simulink model "gm_pmsm_fpga_slrt"  (R2020b)
settings: Solver=FixedStepDiscrete  StartTime=0.0  StopTime=5  FixedStep=1e-5  RelTol=1e-3
PostLoadFcn:
  | try
  | cell = struct2cell(dir(fullfile(speedgoatroot_hdlb, 'hdlsrc', 'pwm', '*.vhd')));
  | addSourceFiles = strjoin(fullfile(cell(2,:),cell(1,:)), ';');
  | hdlset_param('pwm_example_hdlc/DUT PWM and CAP', 'IPCoreAdditionalFiles', addSourceFiles);
  | end
InitFcn:
  | Ts=50e-6;     %simulation time step
  | kp = 1e-4;   %proportional gain
  | ki =0.01e-1;     %integral gain
  | fsw = 1e3;     %switching frequency
undefined symbols (not defined in the file): DiscIntNeverNeededParam, FPGA, IO334, pmsm_fpga
libraries: speedgoatlib_hdlCoder_IO3xx x11, powerlib x9, powerlib_meascontrol x6, quadrature_cpulib x1, slrealtimeutilitieslib x1, pwm_cpulib x1, eeQuadratureDecoder x1, simulink x1, mcbplantlib x1
settings Model: ModifiedByFormat=Speedgoat GmbH  SimulationMode=external  Creator=Speedgoat GmbH  LastModifiedBy=Speedgoat GmbH
settings SolverCC: ConcurrentTasks=on  PositivePriorityOrder=on
settings DataIOCC: LimitDataPoints=on  SaveFormat=Array  ReturnWorkspaceOutputs=off
settings OptimizationCC: BlockReduction=off  ConditionallyExecuteInputs=off  DefaultParameterBehavior=Inlined  OptimizeBlockIOStorage=off
settings DebuggingCC: AlgebraicLoopMsg=error  UnderspecifiedInitializationDetection=Classic  MergeDetectMultiDrivingBlocksExec=none  SolverPrmCheckMsg=warning  InheritedTsInSrcMsg=none  SingleTaskRateTransMsg=error  TasksWithSamePriorityMsg=none  ParameterPrecisionLossMsg=none  PregeneratedLibrarySubsystemCodeDiagnostic=none  SFUnexpectedBacktrackingDiag=warning  SFNoUnconditionalDefaultTransitionDiag=warning  SFExecutionAtInitializationDiag=none  ArithmeticOperatorsInVariantConditions=warning
settings HardwareCC: ProdBitPerLong=64  ProdLongLongMode=on  ProdHWDeviceType=Intel->x86-64 (Linux 64)
settings ModelReferenceCC: PropagateSignalLabelsOutOfModel=off
settings SFSimCC: SimUseLocalCustomCode=off  CustomCodeUndefinedFunction=UseInterfaceOnly
settings RTWCC: Description=Simulink Real-Time  SystemTargetFile=slrealtime.tlc  TemplateMakefile=slrealtime_default_tmf  RTWUseLocalCustomCode=off  Toolchain=Simulink Real-Time Toolchain  BuildConfiguration=Faster Runs  CodeExecutionProfiling=on  TargetLang=C++
settings CodeAppCC: StateflowObjectComments=on
settings ConfigComp: CovMetricSettings=dw  CovSaveCumulativeToWorkspaceVar=on  CovSaveSingleToWorkspaceVar=on  CovExternalEMLEnable=off

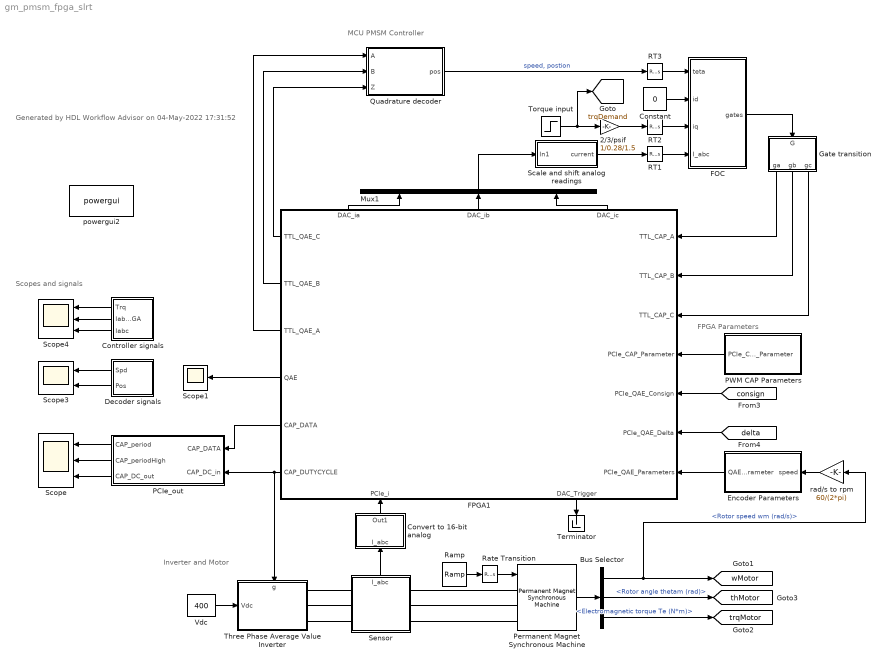
== system gm_pmsm_fpga_slrt ==
  note: Generated by HDL Workflow Advisor on 04-May-2022 17:31:52
  note: FPGA Parameters
  note: Inverter and Motor
  note: MCU PMSM Controller
  note: Scopes and signals
  2/3/psif : Gain  Gain=1/0.28/1.5  SaturateOnIntegerOverflow=on  OutDataTypeStr=Inherit: Same as input  ParamDataTypeStr=Inherit: Same as input
  Bus Selector : BusSelector  OutputSignals=Rotor speed wm (rad/s),Rotor angle thetam (rad),Electromagnetic torque Te (N*m)
  Constant : Constant  Value=0  SampleTime=-1
  Controller signals : Subsystem
  Convert to 16-bit analog : Subsystem
  Decoder signals : Subsystem
  Encoder Parameters : Subsystem
  FOC : Subsystem
  FPGA1 : Subsystem  mask(Speedgoat IO334-325k Interface Block){module_id=1, slot=-1, ts=-1, OutputRange=Auto (same as ADC), PullRPort0=pull-up 3.3V, VioPort0=3.3V, PullRPort1=pull-up 3.3V, VioPort1=3.3V, PullRPort2=pull-up 3.3V, VioPort2=3.3V, PullRPort3=pull-up 3.3V, VioPort3=3.3V, PullRPort4=pull-up 3.3V, VioPort4=3.3V, PullRPort5=pull-up 3.3V, VioPort5=3.3V, PullRPort6=pull-up 3.3V, VioPort6=3.3V, FpgaFreq=100}
      mask prompts: module_id "FPGA Module Identifier:"; slot "PCI slot (-1: autosearch):"; ts "Sample time:"; OutputRange "DAC Voltage Range:"; PullRPort0 "pull resistor"; VioPort0 "I/O voltage"; PullRPort1 "pull resistor"; VioPort1 "I/O voltage"; PullRPort2 "pull resistor"; VioPort2 "I/O voltage"; PullRPort3 "pull resistor"; VioPort3 "I/O voltage"; PullRPort4 "pull resistor"; VioPort4 "I/O voltage"; PullRPort5 "pull resistor"; VioPort5 "I/O voltage"; PullRPort6 "pull resistor"; VioPort6 "I/O voltage"; FpgaFreq "FPGA Frequency [MHz]"
      mask help: Simulink Real-Time Interface Block for Speedgoat IO334-325k.
      mask init:
      | hdlslrt.backend.mfpgaparameters;
      settings: PortSchema="{\"entries\":[{\"content\":{\"sides\":[{\"content\":{\"connectorIds\":[\"Out5\",\"Out6\",\"Out7\",\"Out8\",\"Out9\",\"Out10\"]},\"type\":\"ConnectorPlacement.EquallySpacedRectSide\",\"uuid\":\"34ddc533-e92e-4f84-ab54-56ee31c34ed5\"},{\"content\":{\"connectorIds\":[\"In2\",\"In3\",\"In4\",\"In5\",\"In6\",\"In7\",\"In8\"],\"side\":\"RIGHT\"},\"type\":\"ConnectorPlacement.EquallySpacedRectSide\",\"uuid\":\"fc43732f-8b85-47c9-af73-b87840a05fb5\"},{\"content\":{\"connectorIds\":[\"Out2\",\"Out3\",\"Out4\"],\"side\":\"TOP\"},\"type\":\"ConnectorPlacement.EquallySpacedRectSide\",\"uuid\":\"bf663b9c-33b6-4726-afdb-56df835214b8\"},{\"content\":{\"connectorIds\":[\"In1\",\"Out1\"],\"side\":\"BOTTOM\"},\"type\":\"ConnectorPlacement.EquallySpacedRectSide\",\"uuid\":\"04fbffa8-14ef-4425-a219-a420a37a7cbf\"},{\"content\":{\"connectorIds\":[],\"side\":\"HIDDEN\"},\"type\":\"ConnectorPlacement.EquallySpacedRectSide\",\"uuid\":\"ed9b2637-afe7-435a-b994-99eac90c9c32\"}]},\"type\":\"ConnectorPlacement.EquallySpacedConnector\",\"uuid\":\"b4b9272a-3f4d-4e79-a573-4a3ad4933ba9\"}],\"packageUris\":[\"http://schema.mathworks.com/mf0/Connector/R2020b\"],\"version\":\"1.0\"}"
      mask Help: eval('speedgoatdoc_hdlc')
      mask TypeOptions OutputRange: IO334 DAC Setup/OutputRange
      mask TypeOptions PullRPort0: Port Settings -2x/PullRPort0
      mask Callback PullRPort0: sg_fpga_HDLCoder_io3xx_2x_m(2)
      mask TypeOptions VioPort0: Port Settings -2x/VioPort0
      mask Callback VioPort0: sg_fpga_HDLCoder_io3xx_2x_m(2)
      mask TypeOptions PullRPort1: Port Settings -2x/PullRPort1
      mask Callback PullRPort1: sg_fpga_HDLCoder_io3xx_2x_m(2)
      mask TypeOptions VioPort1: Port Settings -2x/VioPort1
      mask Callback VioPort1: sg_fpga_HDLCoder_io3xx_2x_m(2)
      mask TypeOptions PullRPort2: Port Settings -2x/PullRPort2
      mask Callback PullRPort2: sg_fpga_HDLCoder_io3xx_2x_m(2)
      mask TypeOptions VioPort2: Port Settings -2x/VioPort2
      mask Callback VioPort2: sg_fpga_HDLCoder_io3xx_2x_m(2)
      mask TypeOptions PullRPort3: Port Settings -2x/PullRPort3
      mask Callback PullRPort3: sg_fpga_HDLCoder_io3xx_2x_m(2)
      mask TypeOptions VioPort3: Port Settings -2x/VioPort3
      mask Callback VioPort3: sg_fpga_HDLCoder_io3xx_2x_m(2)
      mask TypeOptions PullRPort4: Port Settings -2x/PullRPort4
      mask Callback PullRPort4: sg_fpga_HDLCoder_io3xx_2x_m(2)
      mask TypeOptions VioPort4: Port Settings -2x/VioPort4
      mask Callback VioPort4: sg_fpga_HDLCoder_io3xx_2x_m(2)
      mask TypeOptions PullRPort5: Port Settings -2x/PullRPort5
      mask Callback PullRPort5: sg_fpga_HDLCoder_io3xx_2x_m(2)
      mask TypeOptions VioPort5: Port Settings -2x/VioPort5
      mask Callback VioPort5: sg_fpga_HDLCoder_io3xx_2x_m(2)
      mask TypeOptions PullRPort6: Port Settings -2x/PullRPort6
      mask Callback PullRPort6: sg_fpga_HDLCoder_io3xx_2x_m(2)
      mask TypeOptions VioPort6: Port Settings -2x/VioPort6
      mask Callback VioPort6: sg_fpga_HDLCoder_io3xx_2x_m(2)
      mask DialogControl AnalogOutput Prompt: Analog Output
      mask DialogControl IO33421 Prompt: IO334-21
      mask DialogControl port1 Prompt: Port 1
      mask DialogControl port2 Prompt: Port 2
      mask DialogControl port3 Prompt: Port 3
      mask DialogControl port4 Prompt: Port 4
      mask DialogControl port5 Prompt: Port 5
      mask DialogControl port6 Prompt: Port 6
      mask DialogControl port7 Prompt: Port 7
      mask Display:
      | SetupBlkPath = find_system(gcb, 'LookUnderMasks', 'all', 'FollowLinks', 'on', 'regexp', 'on', 'Name', 'IO3(\d|x){2}\s+Setup' );
      | SetupBlkPath = SetupBlkPath{1};
      | TS = get_param(SetupBlkPath,'timestamp_mcs');
      | disp(sprintf('Speedgoat IO334-325k\nFPGA I/O Module\n\nTimestamp\n%s\n\nReference Design\nVersion 2.1\n\nMatlab R2020b\n\nPCIe Link Width: X4\nRear Plugin: -21\nAurora Mode: None\nAurora Byteswap: true\n', TS))
  Gate transition : Subsystem
  Mux1 : Mux  Inputs=3
  PCIe_out : Subsystem
  PWM CAP Parameters : Subsystem
  Permanent Magnet Synchronous Machine : powerlib/Machines/Permanent Magnet Synchronous Machine  NbPhases=3  FluxDistribution=Sinusoidal  RotorType=Salient-pole  MechanicalLoad=Speed w  PresetModel=No  ShowDetailedParameters=on  MeasurementBus=off  Resistance=0.1  Inductance=8.5e-3  dqInductances="[0.00006  0.00008]*10"  La=0.000395  MachineConstant=Flux linkage established by magnets (V.s)  Flux=0.28  VoltageCst=50.7864  TorqueCst=0.42  Flat=120  Mechanical=[0.0027 0.0004924 1 0]  PolePairs=1  InitialConditions=[0,0, 0,0]  InitialConditions5ph=[0 0 0 0 0 0]  RefAngle=90 degrees behind phase A axis (modified Park)  IterativeDiscreteModel=Trapezoidal non iterative  TsBlock=-1  TsPowergui=0
  Quadrature decoder : Subsystem
  RT1 : RateTransition  OutPortSampleTimeOpt=Inherit  OutPortSampleTime=Ts
  RT2 : RateTransition  OutPortSampleTimeOpt=Inherit  OutPortSampleTime=Ts
  RT3 : RateTransition  OutPortSampleTimeOpt=Inherit  OutPortSampleTime=Ts
  Ramp : simulink/Sources/Ramp  slope=100/2/60*2*pi  start=0  InitialOutput=0
  Rate Transition : RateTransition  OutPortSampleTime=Ts
  Scale and shift analog readings : Subsystem
  Scope : Scope  NumInputPorts=3
  Scope1 : Scope
  Scope3 : Scope  NumInputPorts=2
  Scope4 : Scope  NumInputPorts=3
  Sensor : Subsystem
      settings: PortSchema="{\"entries\":[{\"content\":{\"sides\":[{\"content\":{\"connectorIds\":[\"LConn1\",\"LConn2\",\"LConn3\"]},\"type\":\"ConnectorPlacement.EquallySpacedRectSide\",\"uuid\":\"d3673cf9-f798-4f95-832a-0ee38b3b4235\"},{\"content\":{\"connectorIds\":[\"RConn1\",\"RConn2\",\"RConn3\"],\"side\":\"RIGHT\"},\"type\":\"ConnectorPlacement.EquallySpacedRectSide\",\"uuid\":\"f1c3e6c7-7356-4e8b-bcca-414f2c82a0be\"},{\"content\":{\"connectorIds\":[\"Out1\"],\"side\":\"TOP\"},\"type\":\"ConnectorPlacement.EquallySpacedRectSide\",\"uuid\":\"10e31bf8-a182-46d8-beca-1ec9bb9081e0\"},{\"content\":{\"connectorIds\":[],\"side\":\"HIDDEN\"},\"type\":\"ConnectorPlacement.EquallySpacedRectSide\",\"uuid\":\"21150a95-24d3-4ba1-92b8-5619804d049c\"}]},\"type\":\"ConnectorPlacement.EquallySpacedConnector\",\"uuid\":\"db0d9e3c-2d98-4024-a8e1-7fc9e86b9a02\"}],\"packageUris\":[\"http://schema.mathworks.com/mf0/Connector/R2020b\"],\"version\":\"1.0\"}"
  Terminator : Terminator
  Three Phase Average Value Inverter : Subsystem
      settings: PortSchema="{\"entries\":[{\"content\":{\"sides\":[{\"content\":{\"connectorIds\":[\"In1\"]},\"type\":\"ConnectorPlacement.EquallySpacedRectSide\",\"uuid\":\"bfacb710-2d3a-4e7b-9063-25c8b87226b9\"},{\"content\":{\"connectorIds\":[\"RConn1\",\"RConn2\",\"RConn3\"],\"side\":\"RIGHT\"},\"type\":\"ConnectorPlacement.EquallySpacedRectSide\",\"uuid\":\"a8d38f79-eb95-4afe-ba2f-2842c1cba801\"},{\"content\":{\"connectorIds\":[\"In2\"],\"side\":\"TOP\"},\"type\":\"ConnectorPlacement.EquallySpacedRectSide\",\"uuid\":\"291d9d52-08e6-4456-8afe-095013b7df64\"},{\"content\":{\"connectorIds\":[],\"side\":\"HIDDEN\"},\"type\":\"ConnectorPlacement.EquallySpacedRectSide\",\"uuid\":\"61aa80b0-9b99-474b-ab67-e014373e5595\"}]},\"type\":\"ConnectorPlacement.EquallySpacedConnector\",\"uuid\":\"1232c420-125a-43af-99e1-be04cd6c95a4\"}],\"packageUris\":[\"http://schema.mathworks.com/mf0/Connector/R2020b\"],\"version\":\"1.0\"}"
  Torque input : Step  Time=0.3  After=300  SampleTime=Ts
  Vdc : Constant  Value=400  SampleTime=Ts
  powergui2 : powerlib/powergui  Priority=1  SimulationMode=Discrete  SampleTime=Ts  frequency=60  Iterations=50  frequencyindice=0  Pbase=100e6  ErrMax=1e-4  UnitsV=kV  UnitsW=MW  buscounter=0  FunctionMessages=off  echomessages=off  EnableUseOfTLC=off  CurrentSourceSwitches=off  DisableSnubberDevices=off  DisableRonSwitches=off  DisableVfSwitches=off  DisplayEquations=off  AutomaticDiscreteSolvers=off  SolverType=Tustin/Backward Euler (TBE)  Interpol=off  ExternalGateDelay=off  methode=off  Ts=100  x0status=blocks  SPID=on  SwTol=0  HookPort=off  NonlinearTolerance=1e-4  nMaxIteration=100  ContinueOnMaxIteration=off  RestoreLinks=warning  ResistiveCurrentMeasurement=off  Frange=[0:2:500]  Ylog=off  Xlog=on  ShowGrid=off  save=off  variable=ZData  structure=0  ZoomFFT=off  StartTime=0.0  cycles=1  DisplayStyle=1  fundamental=60  FreqAxis=off  MaxFrequency=1000  frequencyindicesteady=1  RmsSteady=1  display=off
  rad/s to rpm : Gain  Gain=60/(2*pi)
  tag scope: thMotor=global, trqDemand=global, trqMotor=global, wMotor=global
  wires:
  RT3/1 -> FOC/1(teta)
  Bus Selector/3 -> [trqMotor]  "<Electromagnetic torque Te (N*m)>"
  FPGA1/10(CAP_DUTYCYCLE) -> PCIe_out/2(CAP_DC_in), Three Phase Average Value Inverter/2(g)
  FPGA1/7(TTL_QAE_A) -> Quadrature decoder/1(A)
  Ramp/1 -> Rate Transition/1
  PCIe_out/1(CAP_period) -> Scope/1
  Bus Selector/2 -> [thMotor]  "<Rotor angle thetam (rad)>"
  RT1/1 -> FOC/4(I_abc)
  Bus Selector/1 -> rad/s to rpm/1, [wMotor]  "<Rotor speed wm (rad/s)>"
  FPGA1/8(QAE) -> Scope1/1
  Controller signals/2(Iabc_FPGA) -> Scope4/2
  Scale and shift analog readings/1(current) -> RT1/1
  Controller signals/1(Trq) -> Scope4/1
  Decoder signals/1(Spd) -> Scope3/1
  Sensor/1(I_abc) -> Convert to 16-bit analog/1(I_abc)
  RT2/1 -> FOC/3(iq)
  PCIe_out/3(CAP_DC_out) -> Scope/3
  Permanent Magnet Synchronous Machine/1 -> Bus Selector/1
  Torque input/1 -> [trqDemand], 2/3/psif/1
  Convert to 16-bit analog/1(Out1) -> FPGA1/1(PCIe_i)
  FPGA1/3(DAC_ib) -> Mux1/2
  [consign] -> FPGA1/6(PCIe_QAE_Consign)
  FOC/1(gates) -> Gate transition/1(G)
  FPGA1/1(DAC_Trigger) -> Terminator/1
  Mux1/1 -> Scale and shift analog readings/1(In1)
  FPGA1/2(DAC_ia) -> Mux1/1
  [delta] -> FPGA1/7(PCIe_QAE_Delta)
  Constant/1 -> FOC/2(id)
  Gate transition/1(ga) -> FPGA1/2(TTL_CAP_A)
  Vdc/1 -> Three Phase Average Value Inverter/1(Vdc)
  FPGA1/4(DAC_ic) -> Mux1/3
  Controller signals/3(Iabc) -> Scope4/3
  Decoder signals/2(Pos) -> Scope3/2
  Gate transition/2(gb) -> FPGA1/3(TTL_CAP_B)
  FPGA1/6(TTL_QAE_B) -> Quadrature decoder/2(B)
  2/3/psif/1 -> RT2/1
  Quadrature decoder/1(pos) -> RT3/1  "speed, postion"
  Encoder Parameters/1(QAE_parameter) -> FPGA1/8(PCIe_QAE_Parameters)
  FPGA1/5(TTL_QAE_C) -> Quadrature decoder/3(Z)
  PCIe_out/2(CAP_periodHigh) -> Scope/2
  PWM CAP Parameters/1(PCIe_CAP_Parameter) -> FPGA1/5(PCIe_CAP_Parameter)
  rad/s to rpm/1 -> Encoder Parameters/1(speed)
  FPGA1/9(CAP_DATA) -> PCIe_out/1(CAP_DATA)
  Gate transition/3(gc) -> FPGA1/4(TTL_CAP_C)
  Rate Transition/1 -> Permanent Magnet Synchronous Machine/1
  connections:
  Sensor/LConn3 -- Three Phase Average Value Inverter/RConn3
  Permanent Magnet Synchronous Machine/LConn1 -- Sensor/RConn1
  Sensor/LConn2 -- Three Phase Average Value Inverter/RConn2
  Sensor/LConn1 -- Three Phase Average Value Inverter/RConn1
  Permanent Magnet Synchronous Machine/LConn2 -- Sensor/RConn2
  Permanent Magnet Synchronous Machine/LConn3 -- Sensor/RConn3

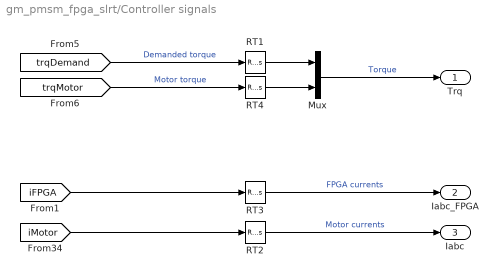
== system gm_pmsm_fpga_slrt/Controller signals ==
  Mux : Mux  Inputs=2
  RT{1..4} (4 alike) : RateTransition  OutPortSampleTime=Ts
  Trq : Outport  VectorParamsAs1DForOutWhenUnconnected=off
  Iabc_FPGA : Outport  Port=2  VectorParamsAs1DForOutWhenUnconnected=off
  Iabc : Outport  Port=3  VectorParamsAs1DForOutWhenUnconnected=off
  wires:
  RT4/1 -> Mux/2
  [trqMotor] -> RT4/1  "Motor torque"
  Mux/1 -> Trq/1  "Torque"
  [iFPGA] -> RT3/1
  RT2/1 -> Iabc/1  "Motor currents"
  [iMotor] -> RT2/1
  RT3/1 -> Iabc_FPGA/1  "FPGA currents"
  RT1/1 -> Mux/1
  [trqDemand] -> RT1/1  "Demanded torque"

== system gm_pmsm_fpga_slrt/Convert to 16-bit analog ==
  I_abc : Inport
  1-D Lookup Table : Lookup_n-D  NumberOfTableDimensions=1  BreakpointsForDimension1=[-2^15, 2^15]  Table=[0, 3.3/10*(2^15-1)]  InternalRulePriority=Speed  RndMeth=Simplest  InputSameDT=on
  Data Type Conversion : DataTypeConversion  OutDataTypeStr=int16
  Gain : Gain  Gain=2^3
  Out1 : Outport
  wires:
  Gain/1 -> 1-D Lookup Table/1
  I_abc/1 -> Gain/1
  1-D Lookup Table/1 -> Data Type Conversion/1
  Data Type Conversion/1 -> Out1/1

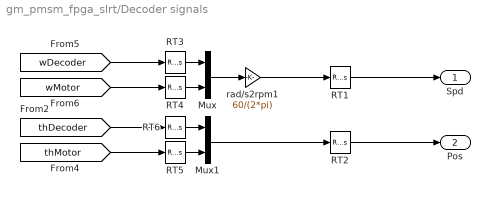
== system gm_pmsm_fpga_slrt/Decoder signals ==
  Mux : Mux  Inputs=2
  Mux1 : Mux  Inputs=2
  RT{1..6} (6 alike) : RateTransition  OutPortSampleTime=Ts
  rad/s2rpm1 : Gain  Gain=60/(2*pi)
  Spd : Outport  VectorParamsAs1DForOutWhenUnconnected=off
  Pos : Outport  Port=2  VectorParamsAs1DForOutWhenUnconnected=off
  wires:
  RT6/1 -> Mux1/1
  RT3/1 -> Mux/1
  rad/s2rpm1/1 -> RT1/1
  RT5/1 -> Mux1/2
  RT4/1 -> Mux/2
  RT2/1 -> Pos/1
  RT1/1 -> Spd/1
  [thMotor] -> RT5/1
  [wMotor] -> RT4/1
  Mux1/1 -> RT2/1
  [thDecoder] -> RT6/1
  Mux/1 -> rad/s2rpm1/1
  [wDecoder] -> RT3/1

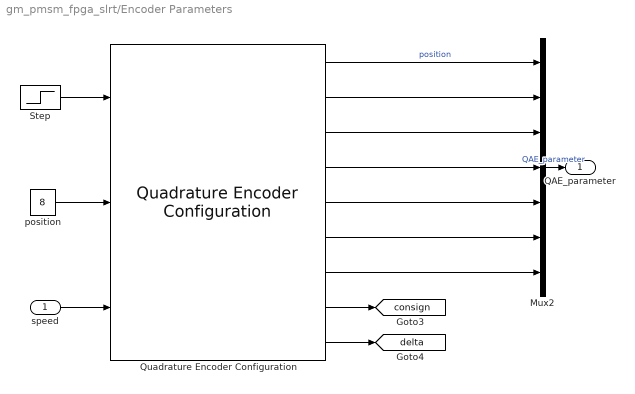
== system gm_pmsm_fpga_slrt/Encoder Parameters ==
  speed : Inport
  Mux2 : Mux  Inputs=7
  Quadrature Encoder Configuration : quadrature_cpulib/Quadrature Encoder Configuration  fpgaFreq=100e6  n_channels=1  numSeg=[512]  phaseAngle=90  initPos=[0]  freeWheel=on
      settings: SourceProductName=Simulink Real-Time: Speedgoat HDL Blockset
  Step : Step  Time=0.002
  position : Constant  Value=8  SampleTime=-1
  QAE_parameter : Outport
  tag scope: consign=global, delta=global
  wires:
  Quadrature Encoder Configuration/3 -> Mux2/3
  Quadrature Encoder Configuration/9 -> [delta]
  Quadrature Encoder Configuration/1 -> Mux2/1  "position"
  Quadrature Encoder Configuration/5 -> Mux2/5
  Quadrature Encoder Configuration/6 -> Mux2/6
  Mux2/1 -> QAE_parameter/1  "QAE_parameter"
  position/1 -> Quadrature Encoder Configuration/2
  Quadrature Encoder Configuration/2 -> Mux2/2
  Quadrature Encoder Configuration/4 -> Mux2/4
  Quadrature Encoder Configuration/7 -> Mux2/7
  Step/1 -> Quadrature Encoder Configuration/1
  Quadrature Encoder Configuration/8 -> [consign]
  speed/1 -> Quadrature Encoder Configuration/3

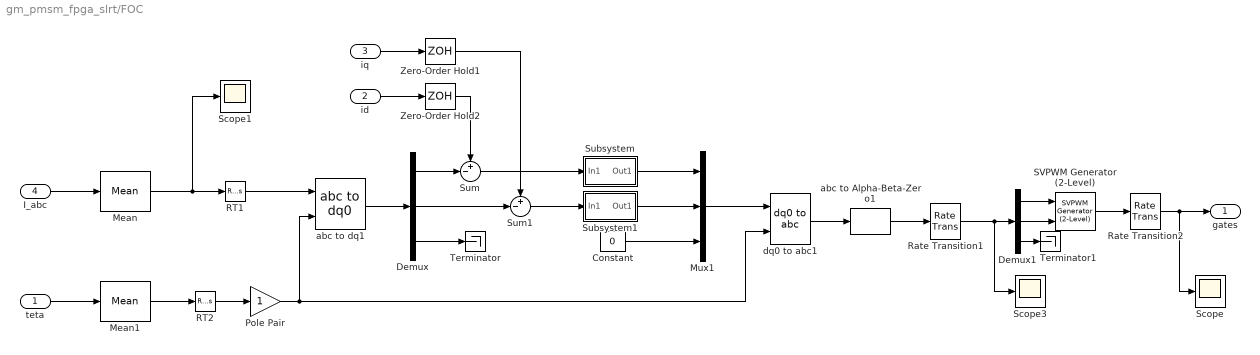
== system gm_pmsm_fpga_slrt/FOC ==
  teta : Inport
  id : Inport  Port=2
  iq : Inport  Port=3
  I_abc : Inport  Port=4
  Constant : Constant  Value=0
  Demux : Demux  Outputs=3
  Demux1 : Demux  Outputs=3
  Mean : powerlib_meascontrol/Measurements/Mean  Freq=fsw  Vinit=0  Ts=Ts
  Mean1 : powerlib_meascontrol/Measurements/Mean  Freq=fsw  Vinit=0  Ts=Ts
  Mux1 : Mux  Inputs=[1 1 1]
  Pole Pair : Gain  SaturateOnIntegerOverflow=on  OutDataTypeStr=Inherit: Same as input  ParamDataTypeStr=Inherit: Same as input
  RT1 : RateTransition  OutPortSampleTimeOpt=Inherit  OutPortSampleTime=Ts
  RT2 : RateTransition  OutPortSampleTimeOpt=Inherit  OutPortSampleTime=Ts
  Rate Transition1 : RateTransition
  Rate Transition2 : RateTransition
  SVPWM Generator (2-Level) : powerlib_meascontrol/Pulse & Signal Generators/SVPWM Generator (2-Level)  InputType=alpha-beta components  SwitchingPattern=Pattern #1  Fc=fsw  ParUref=[0.8 -30 50]  Ts=Ts
      settings: SourceProductBaseCode=PS
  Scope : Scope
  Scope1 : Scope
  Scope3 : Scope
  Subsystem : Subsystem
  Subsystem1 : Subsystem
  Sum : Sum  Inputs=+-|
  Sum1 : Sum  Inputs=+-|
  Terminator : Terminator
  Terminator1 : Terminator
  Zero-Order Hold1 : ZeroOrderHold  SampleTime=1/fsw
  Zero-Order Hold2 : ZeroOrderHold  SampleTime=1/fsw
  abc to Alpha-Beta-Zero1 : powerlib_meascontrol/Transformations/abc to Alpha-Beta-Zero
  abc to dq1 : powerlib_meascontrol/Transformations/abc to dq0  Alignment=90 degrees behind phase A axis
  dq0 to abc1 : powerlib_meascontrol/Transformations/dq0 to abc  Alignment=Aligned with phase A axis
  gates : Outport  VectorParamsAs1DForOutWhenUnconnected=off
  wires:
  abc to dq1/1 -> Demux/1
  Demux/2 -> Sum1/2
  dq0 to abc1/1 -> abc to Alpha-Beta-Zero1/1
  Mean1/1 -> RT2/1
  Pole Pair/1 -> dq0 to abc1/2, abc to dq1/2
  Demux1/1 -> SVPWM Generator (2-Level)/1
  Mean/1 -> RT1/1, Scope1/1
  SVPWM Generator (2-Level)/1 -> Rate Transition2/1
  Demux/3 -> Terminator/1
  iq/1 -> Zero-Order Hold1/1
  Rate Transition2/1 -> gates/1, Scope/1
  id/1 -> Zero-Order Hold2/1
  Demux1/2 -> SVPWM Generator (2-Level)/2
  Mux1/1 -> dq0 to abc1/1
  Subsystem/1(Out1) -> Mux1/1
  Subsystem1/1(Out1) -> Mux1/2
  Constant/1 -> Mux1/3
  teta/1 -> Mean1/1
  Sum1/1 -> Subsystem1/1(In1)
  I_abc/1 -> Mean/1
  Demux/1 -> Sum/2
  Sum/1 -> Subsystem/1(In1)
  Demux1/3 -> Terminator1/1
  Zero-Order Hold1/1 -> Sum1/1
  Zero-Order Hold2/1 -> Sum/1
  abc to Alpha-Beta-Zero1/1 -> Rate Transition1/1
  Rate Transition1/1 -> Demux1/1, Scope3/1
  RT1/1 -> abc to dq1/1
  RT2/1 -> Pole Pair/1

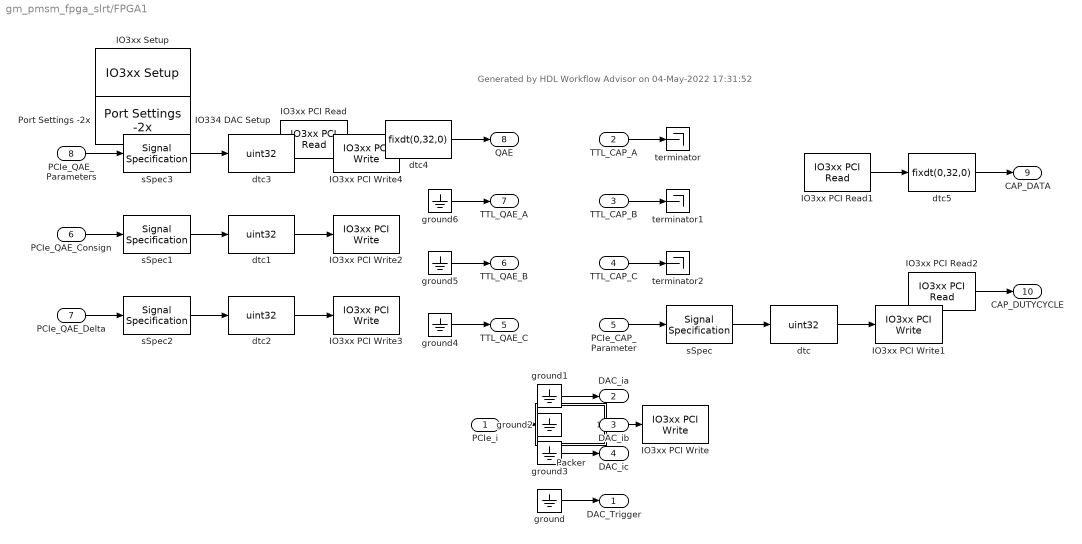
== system gm_pmsm_fpga_slrt/FPGA1 ==
  note: Generated by HDL Workflow Advisor on 04-May-2022 17:31:52
  PCIe_i : Inport  OutDataTypeStr=int16
  TTL_CAP_A : Inport  Port=2
  TTL_CAP_B : Inport  Port=3
  TTL_CAP_C : Inport  Port=4
  PCIe_CAP_Parameter : Inport  Port=5
  PCIe_QAE_Consign : Inport  Port=6
  PCIe_QAE_Delta : Inport  Port=7
  PCIe_QAE_Parameters : Inport  Port=8
  IO334 DAC Setup : speedgoatlib_hdlCoder_IO3xx/IO334 DAC Setup  module_id=module_id  OutputRange=Auto (same as ADC)
  IO3xx PCI Read : speedgoatlib_hdlCoder_IO3xx/IO3xx PCI Read  device_id=1  module_id=module_id  board_type=IO334-325k  port_name=QAE  port_offset=hex2dec('150')  port_type=uint32  port_dim=1  strobe=0  sample_time=ts
  IO3xx PCI Read1 : speedgoatlib_hdlCoder_IO3xx/IO3xx PCI Read  device_id=1  module_id=module_id  board_type=IO334-325k  port_name=CAP_DATA  port_offset=hex2dec('200')  port_type=uint32  port_dim=18  strobe=hex2dec('280')  sample_time=ts
  IO3xx PCI Read2 : speedgoatlib_hdlCoder_IO3xx/IO3xx PCI Read  device_id=1  module_id=module_id  board_type=IO334-325k  port_name=CAP_DUTYCYCLE  port_offset=hex2dec('190')  port_type=single  port_dim=3  strobe=hex2dec('1A0')  sample_time=ts
  IO3xx PCI Write : speedgoatlib_hdlCoder_IO3xx/IO3xx PCI Write  device_id=1  module_id=module_id  board_type=IO334-325k  port_name=PCIe_i  port_offset=hex2dec('100')  port_type=uint32  port_dim=2  strobe=hex2dec('108')  sample_time=ts
  IO3xx PCI Write1 : speedgoatlib_hdlCoder_IO3xx/IO3xx PCI Write  device_id=1  module_id=module_id  board_type=IO334-325k  port_name=PCIe_CAP_Parameter  port_offset=hex2dec('120')  port_type=uint32  port_dim=3  strobe=hex2dec('130')  sample_time=ts
  IO3xx PCI Write2 : speedgoatlib_hdlCoder_IO3xx/IO3xx PCI Write  device_id=1  module_id=module_id  board_type=IO334-325k  port_name=PCIe_QAE_Consign  port_offset=hex2dec('140')  port_type=uint32  port_dim=1  strobe=0  sample_time=ts
  IO3xx PCI Write3 : speedgoatlib_hdlCoder_IO3xx/IO3xx PCI Write  device_id=1  module_id=module_id  board_type=IO334-325k  port_name=PCIe_QAE_Delta  port_offset=hex2dec('118')  port_type=uint32  port_dim=1  strobe=0  sample_time=ts
  IO3xx PCI Write4 : speedgoatlib_hdlCoder_IO3xx/IO3xx PCI Write  device_id=1  module_id=module_id  board_type=IO334-325k  port_name=PCIe_QAE_Parameters  port_offset=hex2dec('160')  port_type=uint32  port_dim=7  strobe=hex2dec('180')  sample_time=ts
  IO3xx Setup : speedgoatlib_hdlCoder_IO3xx/IO3xx Setup  mdl_ss_name=pmsm_fpga/FPGA  board_type=IO334-325k  fpga_sync_mode=on  reset_mode=on  device_id=1  module_id=module_id  pci_slot=slot  fpga_mat_file=hdl_prj\hdlsrc\pmsm_fpga\FPGA.mat  timestamp_mcs=05/04/22 17:25:58  timestamp=2205041640  tsreg=hex2dec('8')  bsf_file=FPGA_2205041640.mcs  mcs=0
  Packer : Subsystem
  Port Settings -2x : speedgoatlib_hdlCoder_IO3xx/Port Settings -2x  module_id=module_id  rearIO=-21  PullRPort0=pull-up 3.3V  VioPort0=3.3V  PullRPort1=pull-up 3.3V  VioPort1=3.3V  PullRPort2=pull-up 3.3V  VioPort2=3.3V  PullRPort3=pull-up 3.3V  VioPort3=3.3V  PullRPort4=pull-up 3.3V  VioPort4=3.3V  PullRPort5=pull-up 3.3V  VioPort5=3.3V  PullRPort6=pull-up 3.3V  VioPort6=3.3V
  dtc{,1..3} (4 alike) : DataTypeConversion  OutDataTypeStr=uint32  ConvertRealWorld=Stored Integer (SI)  RndMeth=Zero
  dtc4 : DataTypeConversion  OutDataTypeStr=fixdt(0,32,0)  ConvertRealWorld=Stored Integer (SI)  RndMeth=Zero
  dtc5 : DataTypeConversion  OutDataTypeStr=fixdt(0,32,0)  ConvertRealWorld=Stored Integer (SI)  RndMeth=Zero
  ground{,1..6} (7 alike) : Ground
  sSpec : SignalSpecification  OutDataTypeStr=fixdt(0,32,0)
  sSpec1 : SignalSpecification  OutDataTypeStr=fixdt(0,32,0)
  sSpec2 : SignalSpecification  OutDataTypeStr=fixdt(1,32,0)
  sSpec3 : SignalSpecification  OutDataTypeStr=fixdt(0,32,0)
  terminator : Terminator
  terminator1 : Terminator
  terminator2 : Terminator
  DAC_Trigger : Outport
  DAC_ia : Outport  Port=2
  DAC_ib : Outport  Port=3
  DAC_ic : Outport  Port=4
  TTL_QAE_C : Outport  Port=5
  TTL_QAE_B : Outport  Port=6
  TTL_QAE_A : Outport  Port=7
  QAE : Outport  Port=8
  CAP_DATA : Outport  Port=9
  CAP_DUTYCYCLE : Outport  Port=10
  wires:
  PCIe_i/1 -> Packer/1(unpacked)
  Packer/1(packed) -> IO3xx PCI Write/1
  TTL_CAP_A/1 -> terminator/1
  TTL_CAP_B/1 -> terminator1/1
  TTL_CAP_C/1 -> terminator2/1
  PCIe_CAP_Parameter/1 -> sSpec/1
  sSpec/1 -> dtc/1
  dtc/1 -> IO3xx PCI Write1/1
  PCIe_QAE_Consign/1 -> sSpec1/1
  sSpec1/1 -> dtc1/1
  dtc1/1 -> IO3xx PCI Write2/1
  PCIe_QAE_Delta/1 -> sSpec2/1
  sSpec2/1 -> dtc2/1
  dtc2/1 -> IO3xx PCI Write3/1
  PCIe_QAE_Parameters/1 -> sSpec3/1
  sSpec3/1 -> dtc3/1
  dtc3/1 -> IO3xx PCI Write4/1
  ground/1 -> DAC_Trigger/1
  ground1/1 -> DAC_ia/1
  ground2/1 -> DAC_ib/1
  ground3/1 -> DAC_ic/1
  ground4/1 -> TTL_QAE_C/1
  ground5/1 -> TTL_QAE_B/1
  ground6/1 -> TTL_QAE_A/1
  dtc4/1 -> QAE/1
  IO3xx PCI Read/1 -> dtc4/1
  dtc5/1 -> CAP_DATA/1
  IO3xx PCI Read1/1 -> dtc5/1
  IO3xx PCI Read2/1 -> CAP_DUTYCYCLE/1

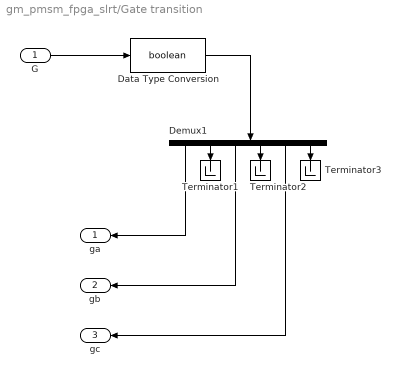
== system gm_pmsm_fpga_slrt/Gate transition ==
  G : Inport
  Data Type Conversion : DataTypeConversion  OutDataTypeStr=boolean
  Demux1 : Demux  Outputs=6
  Terminator1 : Terminator
  Terminator2 : Terminator
  Terminator3 : Terminator
  ga : Outport
  gb : Outport  Port=2
  gc : Outport  Port=3
  wires:
  Demux1/5 -> gc/1
  Demux1/3 -> gb/1
  Demux1/1 -> ga/1
  Demux1/4 -> Terminator2/1
  G/1 -> Data Type Conversion/1
  Demux1/6 -> Terminator3/1
  Demux1/2 -> Terminator1/1
  Data Type Conversion/1 -> Demux1/1

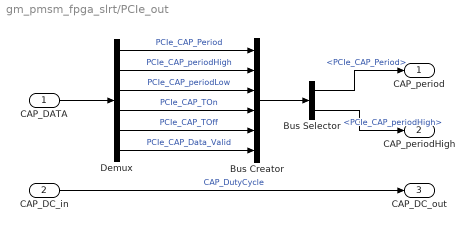
== system gm_pmsm_fpga_slrt/PCIe_out ==
  CAP_DATA : Inport
  CAP_DC_in : Inport  Port=2
  Bus Creator : BusCreator  Inputs=6
  Bus Selector : BusSelector  OutputSignals=PCIe_CAP_Period,PCIe_CAP_periodHigh
  Demux : Demux  Outputs=6
  CAP_period : Outport
  CAP_periodHigh : Outport  Port=2
  CAP_DC_out : Outport  Port=3
  wires:
  CAP_DATA/1 -> Demux/1
  Demux/5 -> Bus Creator/5  "PCIe_CAP_TOff"
  Demux/1 -> Bus Creator/1  "PCIe_CAP_Period"
  Bus Creator/1 -> Bus Selector/1
  Demux/4 -> Bus Creator/4  "PCIe_CAP_TOn"
  Demux/2 -> Bus Creator/2  "PCIe_CAP_periodHigh"
  Demux/3 -> Bus Creator/3  "PCIe_CAP_periodLow"
  Demux/6 -> Bus Creator/6  "PCIe_CAP_Data_Valid"
  Bus Selector/1 -> CAP_period/1  "<PCIe_CAP_Period>"
  Bus Selector/2 -> CAP_periodHigh/1  "<PCIe_CAP_periodHigh>"
  CAP_DC_in/1 -> CAP_DC_out/1  "CAP_DutyCycle"

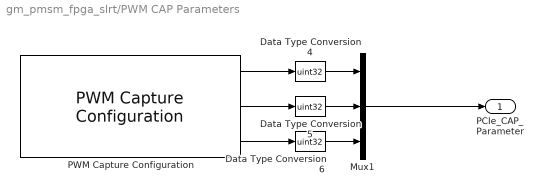
== system gm_pmsm_fpga_slrt/PWM CAP Parameters ==
  Data Type Conversion4 : DataTypeConversion  OutDataTypeStr=uint32
  Data Type Conversion5 : DataTypeConversion  OutDataTypeStr=uint32
  Data Type Conversion6 : DataTypeConversion  OutDataTypeStr=uint32
  Mux1 : Mux  Inputs=3
  PWM Capture Configuration : pwm_cpulib/PWM Capture Configuration  FPGA_freq=100e6  n_channels=1  captureMode=High transitions triggered  captureTimeout=0  PWM_pattern_en=off
      settings: SourceProductName=Simulink Real-Time: Speedgoat HDL Blockset
  PCIe_CAP_Parameter : Outport
  wires:
  PWM Capture Configuration/1 -> Data Type Conversion4/1
  Mux1/1 -> PCIe_CAP_Parameter/1
  PWM Capture Configuration/3 -> Data Type Conversion6/1
  Data Type Conversion4/1 -> Mux1/1
  Data Type Conversion5/1 -> Mux1/2
  Data Type Conversion6/1 -> Mux1/3
  PWM Capture Configuration/2 -> Data Type Conversion5/1

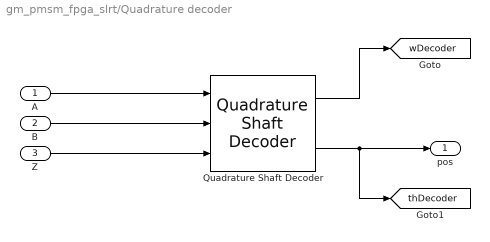
== system gm_pmsm_fpga_slrt/Quadrature decoder ==
  A : Inport
  B : Inport  Port=2
  Z : Inport  Port=3
  Quadrature Shaft Decoder : eeQuadratureDecoder/Quadrature Shaft Decoder  NPulse=256  Ts=-1
      settings: SourceProductBaseCode=PS
  pos : Outport
  tag scope: thDecoder=global, wDecoder=global
  wires:
  A/1 -> Quadrature Shaft Decoder/1
  Quadrature Shaft Decoder/2 -> [thDecoder], pos/1
  Quadrature Shaft Decoder/1 -> [wDecoder]
  B/1 -> Quadrature Shaft Decoder/2
  Z/1 -> Quadrature Shaft Decoder/3

== system gm_pmsm_fpga_slrt/Scale and shift analog readings ==
  In1 : Inport
  1-D Lookup Table : Lookup_n-D  NumberOfTableDimensions=1  BreakpointsForDimension1=[0, 3.3/10*(2^15-1)]  Table=[-2^15, 2^15-1]  InternalRulePriority=Speed  RndMeth=Simplest  InputSameDT=on
  Data Type Conversion : DataTypeConversion  OutDataTypeStr=double
  Scale to max range : Gain  Gain=2^-3
  current : Outport
  tag scope: iFPGA=global
  wires:
  Scale to max range/1 -> [iFPGA], current/1  "current"
  In1/1 -> Data Type Conversion/1
  1-D Lookup Table/1 -> Scale to max range/1
  Data Type Conversion/1 -> 1-D Lookup Table/1

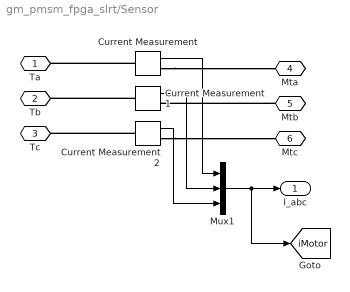
== system gm_pmsm_fpga_slrt/Sensor ==
  Current Measurement : powerlib/Measurements/Current Measurement  PhasorSimulation=off  OutputType=Complex  PSBequivalent=0
  Current Measurement1 : powerlib/Measurements/Current Measurement  PhasorSimulation=off  OutputType=Complex  PSBequivalent=0
  Current Measurement2 : powerlib/Measurements/Current Measurement  PhasorSimulation=off  OutputType=Complex  PSBequivalent=0
  Mux1 : Mux  Inputs=3
  Ta : PMIOPort  Side=Left
  Tb : PMIOPort  Port=2  Side=Left
  Tc : PMIOPort  Port=3  Side=Left
  Mta : PMIOPort  Port=4  Side=Right
  Mtb : PMIOPort  Port=5  Side=Right
  Mtc : PMIOPort  Port=6  Side=Right
  I_abc : Outport  VectorParamsAs1DForOutWhenUnconnected=off
  tag scope: iMotor=global
  wires:
  Current Measurement1/1 -> Mux1/2
  Current Measurement/1 -> Mux1/1
  Current Measurement2/1 -> Mux1/3
  Mux1/1 -> [iMotor], I_abc/1
  connections:
  Mtb/RConn1 -- Current Measurement1/RConn1
  Current Measurement1/LConn1 -- Tb/RConn1
  Current Measurement/RConn1 -- Mta/RConn1
  Current Measurement/LConn1 -- Ta/RConn1
  Current Measurement2/LConn1 -- Tc/RConn1
  Current Measurement2/RConn1 -- Mtc/RConn1

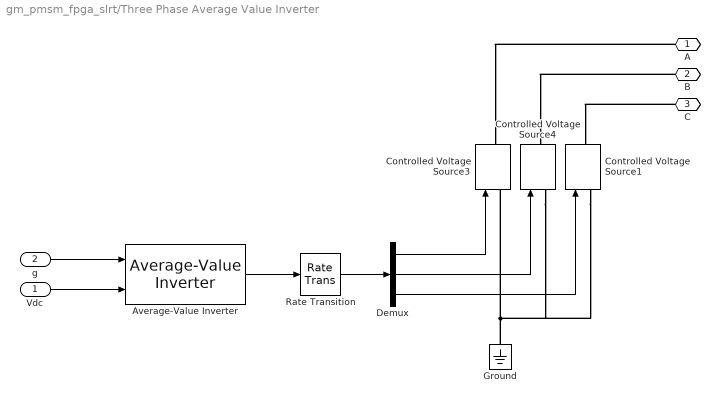
== system gm_pmsm_fpga_slrt/Three Phase Average Value Inverter ==
  Vdc : Inport
  g : Inport  Port=2
  Average-Value Inverter : mcbplantlib/Average-Value Inverter
  Controlled Voltage Source1 : powerlib/Electrical Sources/Controlled Voltage Source  Initialize=on  Source_Type=AC  Amplitude=0  Phase=0  Frequency=0  Measurements=None
  Controlled Voltage Source3 : powerlib/Electrical Sources/Controlled Voltage Source  Initialize=on  Source_Type=AC  Amplitude=0  Phase=0  Frequency=0  Measurements=None
  Controlled Voltage Source4 : powerlib/Electrical Sources/Controlled Voltage Source  Initialize=on  Source_Type=AC  Amplitude=0  Phase=0  Frequency=0  Measurements=None
  Demux : Demux  Outputs=3
  Ground : powerlib/Elements/Ground  LConnTagsString=a
  Rate Transition : RateTransition
  A : PMIOPort  Tag=PMCPort  Side=Right
  B : PMIOPort  Tag=PMCPort  Port=2  Side=Right
  C : PMIOPort  Tag=PMCPort  Port=3  Side=Right
  wires:
  Average-Value Inverter/1 -> Rate Transition/1
  Rate Transition/1 -> Demux/1
  g/1 -> Average-Value Inverter/1
  Demux/1 -> Controlled Voltage Source3/1
  Demux/2 -> Controlled Voltage Source4/1
  Vdc/1 -> Average-Value Inverter/2
  Demux/3 -> Controlled Voltage Source1/1
  connections:
  Ground/LConn1 -- Controlled Voltage Source1/LConn1 -- Controlled Voltage Source4/LConn1 -- Controlled Voltage Source3/LConn1
  C/RConn1 -- Controlled Voltage Source1/RConn1
  B/RConn1 -- Controlled Voltage Source4/RConn1
  A/RConn1 -- Controlled Voltage Source3/RConn1

== system gm_pmsm_fpga_slrt/FOC/Subsystem ==
  In1 : Inport
  Discrete-Time Integrator : DiscreteIntegrator  gainval=ki  SampleTime=-1  LimitOutput=on  UpperSaturationLimit=1  LowerSaturationLimit=-1  ICPrevOutput=DiscIntNeverNeededParam  ICPrevScaledInput=DiscIntNeverNeededParam
  Gain2 : Gain  Gain=kp  SaturateOnIntegerOverflow=on  OutDataTypeStr=Inherit: Same as input  ParamDataTypeStr=Inherit: Same as input
  Sum2 : Sum  Inputs=++|
  Out1 : Outport  VectorParamsAs1DForOutWhenUnconnected=off
  wires:
  Gain2/1 -> Sum2/2
  In1/1 -> Discrete-Time Integrator/1, Gain2/1
  Sum2/1 -> Out1/1
  Discrete-Time Integrator/1 -> Sum2/1

== system gm_pmsm_fpga_slrt/FOC/Subsystem1 ==
  In1 : Inport
  Discrete-Time Integrator : DiscreteIntegrator  gainval=ki  SampleTime=-1  LimitOutput=on  UpperSaturationLimit=1  LowerSaturationLimit=-1  ICPrevOutput=DiscIntNeverNeededParam  ICPrevScaledInput=DiscIntNeverNeededParam
  Gain2 : Gain  Gain=kp  SaturateOnIntegerOverflow=on  OutDataTypeStr=Inherit: Same as input  ParamDataTypeStr=Inherit: Same as input
  Sum2 : Sum  Inputs=++|
  Out1 : Outport  VectorParamsAs1DForOutWhenUnconnected=off
  wires:
  Gain2/1 -> Sum2/2
  In1/1 -> Discrete-Time Integrator/1, Gain2/1
  Sum2/1 -> Out1/1
  Discrete-Time Integrator/1 -> Sum2/1

== system gm_pmsm_fpga_slrt/FPGA1/Packer ==
  unpacked : Inport
  pack : slrealtimeutilitieslib/Bit Packing  MaskBitPatterns={[0:15 16:31 32:47 ]}  MaskPackDataType=uint32  MaskPackDataSize=2
      settings: SourceProductBaseCode=XP
  sSpec : SignalSpecification  OutDataTypeStr=fixdt(1,16,0)
  upconvert : DataTypeConversion  OutDataTypeStr=uint16  ConvertRealWorld=Stored Integer (SI)  RndMeth=Zero
  packed : Outport
  wires:
  unpacked/1 -> sSpec/1
  sSpec/1 -> upconvert/1
  upconvert/1 -> pack/1
  pack/1 -> packed/1
